simulink model "simulation_upgrade"  (R2024b)
settings: Solver=ode1be  StartTime=0.0  StopTime=10  FixedStep=0.001  RelTol=1e-3
model workspace (MAT data in the model file):
  AMP = 1
  FREQ = 1
  i_abc = 1
values from neighbouring files (symbols this model uses):
  v_WLTP = [0 0 0 0 0 0 0 0 0 0 0 0 ... (180001 elements, 1x180001)]    [v_WLTP.mat]
undefined symbols (not defined in the file or in its folder): A, a_sig, b_sig, C1, C2, C3, Cd, CG_z, downshift, Drive_wheel, Driveshaft, f_blend, f_OVD, fo, front_seat_dist, fs, g, Gearbox, i, i_sig, Inclination, Inertia, Jr2, K, m, M_curve_1, M_curve_2, m_driver, M_N_1, M_N_2, mi_c, mi_s, Mode, N_clutch, n_curve_1, n_curve_2, n_driver, n_max_1, n_max_2, n_shift, n_surfaces, Pl, Planetary, r_eq_clutch, r_geom, r_wheel, rho, Shaft, shift_time, sigma0, sigma1, sigma2, slope_angle, Stage1, Stage2, Stage3, upshift, v0, vel_wind, vs ... (+5)
libraries: simulink x29, slpidlib x3
(part 8 of 9)

== system simulation_upgrade/DRIVETRAIN/Transmission/Gearbox/DCT/Clutch1 ==
  M_in : Inport
  clutch1 : Inport  Port=2
  clutch2 : Inport  Port=3
  w_out1 : Inport  Port=4
  w_out2 : Inport  Port=5
  Clutch1 : Subsystem
      settings: PortSchema="{\"entries\":[{\"content\":{\"sides\":[{\"content\":{\"connectorIds\":[\"In1\"]},\"type\":\"ConnectorPlacement.EquallySpacedRectSide\",\"uuid\":\"a26f5a32-9f9c-4306-b7a8-6355090a4a86\"},{\"content\":{\"connectorIds\":[\"Out1\"],\"side\":\"RIGHT\"},\"type\":\"ConnectorPlacement.EquallySpacedRectSide\",\"uuid\":\"4fa489e2-cd1d-4a36-b0cb-261100046200\"},{\"content\":{\"connectorIds\":[\"In2\"],\"side\":\"TOP\"},\"type\":\"ConnectorPlacement.EquallySpacedRectSide\",\"uuid\":\"0e05a540-d6e3-4351-9a32-83f6c32571ff\"}]},\"type\":\"ConnectorPlacement.EquallySpacedConnector\",\"uuid\":\"492e0439-728a-4999-b29b-e2639b0e762e\"}],\"packageUris\":[\"http://schema.mathworks.com/mf0/Connector/R2020b\"],\"version\":\"1.0\"}"
  Clutch2 : Subsystem
      settings: PortSchema="{\"entries\":[{\"content\":{\"sides\":[{\"content\":{\"connectorIds\":[\"In1\"]},\"type\":\"ConnectorPlacement.EquallySpacedRectSide\",\"uuid\":\"a26f5a32-9f9c-4306-b7a8-6355090a4a86\"},{\"content\":{\"connectorIds\":[\"Out1\"],\"side\":\"RIGHT\"},\"type\":\"ConnectorPlacement.EquallySpacedRectSide\",\"uuid\":\"4fa489e2-cd1d-4a36-b0cb-261100046200\"},{\"content\":{\"connectorIds\":[\"In2\"],\"side\":\"TOP\"},\"type\":\"ConnectorPlacement.EquallySpacedRectSide\",\"uuid\":\"0e05a540-d6e3-4351-9a32-83f6c32571ff\"}]},\"type\":\"ConnectorPlacement.EquallySpacedConnector\",\"uuid\":\"492e0439-728a-4999-b29b-e2639b0e762e\"}],\"packageUris\":[\"http://schema.mathworks.com/mf0/Connector/R2020b\"],\"version\":\"1.0\"}"
  Constant1 : Constant  Value=2*Shaft.J+Stage2.Spur11.J+Stage2.Spur21.J
  Constant2 : Constant  Value=N_clutch*mi_s*r_eq_clutch*n_surfaces
  Divide : Product  Inputs=*/
  Integrator : Integrator
  Scope : Scope  NumInputPorts=3
  Scope1 : Scope  NumInputPorts=4
  Scope2 : Scope  NumInputPorts=3
  Scope4 : Scope  NumInputPorts=2
  Sum1 : Sum  Inputs=-+-
  Sum2 : Sum  Inputs=|+-
  Sum3 : Sum  Inputs=-+|
  M_clutch1 : Outport
  M_clutch2 : Outport  Port=2
  w_in : Outport  Port=3
  wires:
  Constant2/1 -> Scope1/4
  Sum3/1 -> Clutch1/1(delta_w), Scope2/1  "delta_w1"
  M_in/1 -> Sum1/2, Scope1/3
  w_out1/1 -> Scope2/3, Sum3/1
  Clutch1/1(M_clutch) -> M_clutch1/1, Scope1/1, Sum1/1
  Sum1/1 -> Scope4/1, Divide/1
  clutch1/1 -> Clutch1/2(" ")
  Integrator/1 -> w_in/1, Scope/2, Sum2/1, Scope2/2, Sum3/2
  Clutch2/1(M_clutch) -> Scope1/2, Sum1/3, M_clutch2/1
  clutch2/1 -> Clutch2/2(" ")
  w_out2/1 -> Scope/1, Sum2/2
  Sum2/1 -> Clutch2/1(delta_w), Scope/3  "delta_w2"
  Divide/1 -> Scope4/2, Integrator/1
  Constant1/1 -> Divide/2

== system simulation_upgrade/DRIVETRAIN/Transmission/Gearbox/DCT/Stage_2.1 ==
  note: 1) Add Subsystem or Model blocks as valid variant choices.
      | 2) You cannot connect blocks at this level. At simulation, connectivity is automatically
      | determined, based on the active variant and port name matching.
  Torque_in : Inport
  Speed_fdbk : Inport  Port=2
  Nothing : Subsystem  VariantControl=Stage2.Type == 0
  Spur : Subsystem  VariantControl=Stage2.Type == 1
  Torque_out : Outport
  Speed_out : Outport  Port=2

== system simulation_upgrade/DRIVETRAIN/Transmission/Gearbox/DCT/Stage_2.2 ==
  note: 1) Add Subsystem or Model blocks as valid variant choices.
      | 2) You cannot connect blocks at this level. At simulation, connectivity is automatically
      | determined, based on the active variant and port name matching.
  Torque_in : Inport
  Speed_fdbk : Inport  Port=2
  Nothing : Subsystem  VariantControl=Stage2.Type == 0
  Spur : Subsystem  VariantControl=Stage2.Type == 1
  Torque_out : Outport
  Speed_out : Outport  Port=2

== system simulation_upgrade/DRIVETRAIN/Transmission/Gearbox/DCT/Stage_3 ==
  note: 1) Add Subsystem or Model blocks as valid variant choices.
      | 2) You cannot connect blocks at this level. At simulation, connectivity is automatically
      | determined, based on the active variant and port name matching.
  Torque_in : Inport
  Speed_fdbk : Inport  Port=2
  Nothing : Subsystem  VariantControl=Stage3.Type == 0
  Spur : Subsystem  VariantControl=Stage3.Type == 1
  Torque_out : Outport
  Speed_out : Outport  Port=2

== system simulation_upgrade/DRIVETRAIN/Transmission/Gearbox/DCT/Triggered Subsystem ==
  In1 : Inport
  Trigger : TriggerPort  TriggerType=either  VariantControl=(inherit)  InitialTriggerSignalState=zero
  Out1 : Outport
  wires:
  In1/1 -> Out1/1

== system simulation_upgrade/DRIVETRAIN/Transmission/Gearbox/TDT/Shaft ==
  Torque_in : Inport
  Speed_fdbk : Inport  Port=2
  Derivative : Derivative
  Gain3 : Gain  Gain=J
  Sum1 : Sum  Inputs=|+-
  Torque_out : Outport
  phi_dot : Outport  Port=2
  wires:
  Speed_fdbk/1 -> phi_dot/1, Derivative/1
  Sum1/1 -> Torque_out/1
  Derivative/1 -> Gain3/1
  Gain3/1 -> Sum1/2
  Torque_in/1 -> Sum1/1

== system simulation_upgrade/DRIVETRAIN/Transmission/Gearbox/TDT/Spur ==
  Torque_in : Inport
  Speed_fdbk : Inport  Port=2
  Derivative : Derivative
  Derivative1 : Derivative
  Gain : Gain  Gain=i
  Gain2 : Gain  Gain=J2
  Gain3 : Gain  Gain=J1
  Gain4 : Gain  Gain=i
  Sum1 : Sum  Inputs=|+-
  Sum2 : Sum  Inputs=|+-
  Torque_out : Outport
  phi_dot : Outport  Port=2
  wires:
  Gain/1 -> Sum2/1
  Sum2/1 -> Torque_out/1
  Gain3/1 -> Sum1/2
  Torque_in/1 -> Sum1/1
  Gain4/1 -> Derivative1/1, phi_dot/1
  Speed_fdbk/1 -> Gain4/1, Derivative/1
  Gain2/1 -> Sum2/2
  Sum1/1 -> Gain/1
  Derivative1/1 -> Gain3/1
  Derivative/1 -> Gain2/1

== system simulation_upgrade/DRIVETRAIN/Transmission/Gearbox/TDT/Spur2 ==
  Torque_in : Inport
  Speed_fdbk : Inport  Port=2
  Derivative : Derivative
  Derivative1 : Derivative
  Gain : Gain  Gain=i
  Gain2 : Gain  Gain=J2
  Gain3 : Gain  Gain=J1
  Gain4 : Gain  Gain=i
  Sum1 : Sum  Inputs=|+-
  Sum2 : Sum  Inputs=|+-
  Torque_out : Outport
  phi_dot : Outport  Port=2
  wires:
  Derivative/1 -> Gain2/1
  Derivative1/1 -> Gain3/1
  Sum1/1 -> Gain/1
  Gain2/1 -> Sum2/2
  Speed_fdbk/1 -> Derivative/1, Gain4/1
  Gain4/1 -> phi_dot/1, Derivative1/1
  Torque_in/1 -> Sum1/1
  Gain3/1 -> Sum1/2
  Sum2/1 -> Torque_out/1
  Gain/1 -> Sum2/1

== system simulation_upgrade/DRIVETRAIN/Transmission/Gearbox/TDT/Stage_1 ==
  note: 1) Add Subsystem or Model blocks as valid variant choices.
      | 2) You cannot connect blocks at this level. At simulation, connectivity is automatically
      | determined, based on the active variant and port name matching.
  Torque_in : Inport
  Speed_fdbk : Inport  Port=2
  Nothing : Subsystem  VariantControl=Stage1.Type == 0
  Spur : Subsystem  VariantControl=Stage1.Type == 1
  Torque_out : Outport
  Speed_out : Outport  Port=2

== system simulation_upgrade/DRIVETRAIN/Transmission/Gearbox/TDT/Stage_2.1 ==
  note: 1) Add Subsystem or Model blocks as valid variant choices.
      | 2) You cannot connect blocks at this level. At simulation, connectivity is automatically
      | determined, based on the active variant and port name matching.
  Torque_in : Inport
  Speed_fdbk : Inport  Port=2
  Nothing : Subsystem  VariantControl=Stage2.Type == 0
  Spur : Subsystem  VariantControl=Stage2.Type == 1
  Torque_out : Outport
  Speed_out : Outport  Port=2

== system simulation_upgrade/DRIVETRAIN/Transmission/Gearbox/TDT/Stage_2.2 ==
  note: 1) Add Subsystem or Model blocks as valid variant choices.
      | 2) You cannot connect blocks at this level. At simulation, connectivity is automatically
      | determined, based on the active variant and port name matching.
  Torque_in : Inport
  Speed_fdbk : Inport  Port=2
  Nothing : Subsystem  VariantControl=Stage2.Type == 0
  Spur : Subsystem  VariantControl=Stage2.Type == 1
  Torque_out : Outport
  Speed_out : Outport  Port=2

== system simulation_upgrade/DRIVETRAIN/Transmission/Gearbox/TDT/Stage_3 ==
  note: 1) Add Subsystem or Model blocks as valid variant choices.
      | 2) You cannot connect blocks at this level. At simulation, connectivity is automatically
      | determined, based on the active variant and port name matching.
  Torque_in : Inport
  Speed_fdbk : Inport  Port=2
  Nothing : Subsystem  VariantControl=Stage3.Type == 0
  Spur : Subsystem  VariantControl=Stage3.Type == 1
  Torque_out : Outport
  Speed_out : Outport  Port=2

== system simulation_upgrade/DRIVETRAIN/Transmission/Gearbox/TDT/Subsystem ==
  Spur 21 : Inport
  Spur22 : Inport  Port=2
  Multiport Switch : MultiPortSwitch  DataPortOrder=Zero-based contiguous  Inputs=8  zeroidx=on  SaturateOnIntegerOverflow=off  InputSameDT=off
  Multiport Switch1 : MultiPortSwitch  DataPortOrder=Zero-based contiguous  zeroidx=on  SaturateOnIntegerOverflow=off  InputSameDT=off
  Switch : Switch  Criteria=u2 > Threshold  Threshold=1  SaturateOnIntegerOverflow=off  InputSameDT=off
  Switch1 : Switch  Criteria=u2 > Threshold  Threshold=1  SaturateOnIntegerOverflow=off  InputSameDT=off
  Out : Outport
  wires:
  Multiport Switch/1 -> Out/1
  [Gear] -> Multiport Switch1/1
  Spur 21/1 -> Multiport Switch1/3, Switch1/1, Switch/3
  Spur22/1 -> Switch/1, Switch1/3, Multiport Switch1/4
  Multiport Switch1/1 -> Multiport Switch/9, Multiport Switch/8, Multiport Switch/7, Multiport Switch/4, Multiport Switch/3, Multiport Switch/2
  [shifting_stage] -> Multiport Switch/1
  [GearSet] -> Switch/2, Switch1/2
  Switch/1 -> Multiport Switch1/2, Multiport Switch/6
  Switch1/1 -> Multiport Switch/5

== system simulation_upgrade/PANEL/Pretty shot/Transmission /Variant Subsystem/Automated Manual Transmission ==
  " " : Inport
  "  " : Outport

== system simulation_upgrade/PANEL/Pretty shot/Transmission /Variant Subsystem/Automatic Transmission ==
  " " : Inport
  "  " : Outport

== system simulation_upgrade/PANEL/Pretty shot/Transmission /Variant Subsystem/Twin Drive Transmission ==
  " " : Inport
  To Workspace : ToWorkspace  VariableName=v_TDT1  SaveFormat=Timeseries  SampleTime=-1
  To Workspace1 : ToWorkspace  VariableName=acc_TDT1  SaveFormat=Timeseries  SampleTime=-1
  To Workspace2 : ToWorkspace  VariableName=jerk_TDT1  SaveFormat=Timeseries  SampleTime=-1
  "  " : Outport
  wires:
  " "/1 -> "  "/1
  [Speed] -> To Workspace/1
  [acc] -> To Workspace1/1
  [jerk] -> To Workspace2/1

== system simulation_upgrade/CONTROLS/Main Control Unit/AT_MCU/Clutch_Profile/polynomial_s_response/signal_register ==
  signal : Inport
  Trigger : TriggerPort  TriggerType=either  VariantControl=(inherit)  PortDimensions=1
  Memory : Memory  InheritSampleTime=on
  Subtract : Sum  Inputs=+-
  previous_value : Outport
  difference : Outport  Port=2
  wires:
  signal/1 -> Memory/1, Subtract/1
  Memory/1 -> previous_value/1, Subtract/2
  Subtract/1 -> difference/1

== system simulation_upgrade/CONTROLS/Main Control Unit/AT_MCU/Clutch_Profile/polynomial_s_response/time_register ==
  t : Inport
  Trigger : TriggerPort  TriggerType=either  VariantControl=(inherit)  PortDimensions=1
  t0 : Outport
  wires:
  t/1 -> t0/1

== system simulation_upgrade/CONTROLS/Main Control Unit/AT_MCU/Clutch_Profile/polynomial_s_response1/signal_register ==
  signal : Inport
  Trigger : TriggerPort  TriggerType=either  VariantControl=(inherit)  PortDimensions=1
  Memory : Memory  InheritSampleTime=on
  Subtract : Sum  Inputs=+-
  previous_value : Outport
  difference : Outport  Port=2
  wires:
  Subtract/1 -> difference/1
  Memory/1 -> Subtract/2, previous_value/1
  signal/1 -> Subtract/1, Memory/1

== system simulation_upgrade/CONTROLS/Main Control Unit/AT_MCU/Clutch_Profile/polynomial_s_response1/time_register ==
  t : Inport
  Trigger : TriggerPort  TriggerType=either  VariantControl=(inherit)  PortDimensions=1
  t0 : Outport
  wires:
  t/1 -> t0/1

== system simulation_upgrade/CONTROLS/Main Control Unit/AT_MCU/Clutch_Profile/sigmoid_response/signal_register ==
  signal : Inport
  Trigger : TriggerPort  TriggerType=either  VariantControl=(inherit)  PortDimensions=1
  Delay : Delay  DelayLength=1  InputProcessing=Columns as channels (frame based)
  Subtract : Sum  Inputs=+-
  previous_value : Outport
  difference : Outport  Port=2
  wires:
  signal/1 -> Delay/1, Subtract/1
  Delay/1 -> previous_value/1, Subtract/2
  Subtract/1 -> difference/1

== system simulation_upgrade/CONTROLS/Main Control Unit/AT_MCU/Clutch_Profile/sigmoid_response/time_register ==
  t : Inport
  Trigger : TriggerPort  TriggerType=either  VariantControl=(inherit)  PortDimensions=1
  t0 : Outport
  wires:
  t/1 -> t0/1

== system simulation_upgrade/CONTROLS/Main Control Unit/AT_MCU/Clutch_Profile/sigmoid_response1/signal_register ==
  signal : Inport
  Trigger : TriggerPort  TriggerType=either  VariantControl=(inherit)  PortDimensions=1
  Delay : Delay  DelayLength=1  InputProcessing=Columns as channels (frame based)
  Subtract : Sum  Inputs=+-
  previous_value : Outport
  difference : Outport  Port=2
  wires:
  Subtract/1 -> difference/1
  Delay/1 -> Subtract/2, previous_value/1
  signal/1 -> Subtract/1, Delay/1

== system simulation_upgrade/CONTROLS/Main Control Unit/AT_MCU/Clutch_Profile/sigmoid_response1/time_register ==
  t : Inport
  Trigger : TriggerPort  TriggerType=either  VariantControl=(inherit)  PortDimensions=1
  t0 : Outport
  wires:
  t/1 -> t0/1

== system simulation_upgrade/DRIVETRAIN/Transmission/Gearbox/AMT/Clutch/Clutch1 ==
  delta_w : Inport
  " " : Inport  Port=2
  Gain10 : Gain  Gain=r_eq_clutch
  Gain3 : Gain  Gain=r_eq_clutch
  Scope2 : Scope  NumInputPorts=2
  Scope3 : Scope
  Subsystem : Subsystem
      settings: PortSchema="{\"entries\":[{\"content\":{\"sides\":[{\"content\":{\"connectorIds\":[\"In1\"]},\"type\":\"ConnectorPlacement.EquallySpacedRectSide\",\"uuid\":\"0ae2ed28-5be6-4ce0-b87c-2c13a72d1ad0\"},{\"content\":{\"connectorIds\":[\"In2\",\"Out1\"],\"side\":\"RIGHT\"},\"type\":\"ConnectorPlacement.EquallySpacedRectSide\",\"uuid\":\"8d48d664-ebaf-4c3e-be9e-f793543e8061\"},{\"content\":{\"side\":\"TOP\"},\"type\":\"ConnectorPlacement.EquallySpacedRectSide\",\"uuid\":\"2d66836a-de46-4974-a48b-ee2778be1c08\"},{\"content\":{\"side\":\"BOTTOM\"},\"type\":\"ConnectorPlacement.EquallySpacedRectSide\",\"uuid\":\"e232d9f4-6257-4976-8384-26c462ae0041\"}]},\"type\":\"ConnectorPlacement.EquallySpacedConnector\",\"uuid\":\"ae24f926-3a59-4a74-9cf0-af55dcfbad19\"}],\"packageUris\":[\"http://schema.mathworks.com/mf0/Connector/R2020b\"],\"version\":\"1.0\"}"
      mask Display: image('images/Stribeck.png');
  Subsystem1 : Subsystem
      settings: PortSchema="{\"entries\":[{\"content\":{\"sides\":[{\"content\":{\"connectorIds\":[\"In1\",\"In2\"]},\"type\":\"ConnectorPlacement.EquallySpacedRectSide\",\"uuid\":\"9e2cbd08-5b8a-4c75-ae53-c0d295cfe494\"},{\"content\":{\"connectorIds\":[\"Out1\",\"Out2\"],\"side\":\"RIGHT\"},\"type\":\"ConnectorPlacement.EquallySpacedRectSide\",\"uuid\":\"77a3a6f0-22a7-43a6-8d61-33ee07a6a335\"},{\"content\":{\"side\":\"TOP\"},\"type\":\"ConnectorPlacement.EquallySpacedRectSide\",\"uuid\":\"42262743-4dc6-4297-a012-95f629a18d23\"},{\"content\":{\"connectorIds\":[\"In3\"],\"side\":\"BOTTOM\"},\"type\":\"ConnectorPlacement.EquallySpacedRectSide\",\"uuid\":\"a89123f6-acee-411d-93c1-3b5d847486f5\"}]},\"type\":\"ConnectorPlacement.EquallySpacedConnector\",\"uuid\":\"ae5ede95-cba8-4d2e-b0da-ab555bd567a9\"}],\"packageUris\":[\"http://schema.mathworks.com/mf0/Connector/R2020b\"],\"version\":\"1.0\"}"
      mask Display: image('images/z_state.png');
  Subsystem2 : Subsystem
      settings: PortSchema="{\"entries\":[{\"content\":{\"sides\":[{\"content\":{\"connectorIds\":[\"In1\",\"In2\",\"In3\"]},\"type\":\"ConnectorPlacement.EquallySpacedRectSide\",\"uuid\":\"1b79fb4b-1921-4665-8eba-b393f9ea98d6\"},{\"content\":{\"connectorIds\":[\"Out1\"],\"side\":\"RIGHT\"},\"type\":\"ConnectorPlacement.EquallySpacedRectSide\",\"uuid\":\"084d95ac-1716-4b0b-a696-3271535a91cf\"},{\"content\":{\"side\":\"TOP\"},\"type\":\"ConnectorPlacement.EquallySpacedRectSide\",\"uuid\":\"ec91298b-c3b0-4df1-a0b8-53c7de39a879\"},{\"content\":{\"connectorIds\":[\"In4\"],\"side\":\"BOTTOM\"},\"type\":\"ConnectorPlacement.EquallySpacedRectSide\",\"uuid\":\"de14d308-9d82-4371-86bd-ca5ab581d7ed\"}]},\"type\":\"ConnectorPlacement.EquallySpacedConnector\",\"uuid\":\"ce361a1b-48ea-4ff5-b8e2-9f4b10df6d4d\"}],\"packageUris\":[\"http://schema.mathworks.com/mf0/Connector/R2020b\"],\"version\":\"1.0\"}"
      mask Display: image('images/fric_force.png');
  M_clutch : Outport
  wires:
  delta_w/1 -> Gain3/1
  Subsystem1/2(z) -> Scope2/1, Subsystem2/3(z)
  Subsystem1/1(z_dot) -> Scope2/2, Subsystem2/2(z_dot)
  Subsystem2/1(F) -> Gain10/1
  Gain10/1 -> M_clutch/1  "M_clutch"
  Gain3/1 -> Scope3/1, Subsystem2/1(v), Subsystem/2(v), Subsystem1/1(v)  "v"
  " "/1 -> Subsystem2/4(" "), Subsystem1/3(In1), Subsystem/1(N)
  Subsystem/1(g(v)) -> Subsystem1/2(g(v))

== system simulation_upgrade/DRIVETRAIN/Transmission/Gearbox/AMT/Stage_1/Nothing ==
  Torque_in : Inport
  Speed_fdbk : Inport  Port=2
  Torque_out : Outport
  Speed_out : Outport  Port=2
  wires:
  Torque_in/1 -> Torque_out/1
  Speed_fdbk/1 -> Speed_out/1

== system simulation_upgrade/DRIVETRAIN/Transmission/Gearbox/AMT/Stage_1/Spur ==
  Torque_in : Inport
  Speed_fdbk : Inport  Port=2
  Shaft1 : Subsystem  mask{J=Shaft.J}
      mask prompts: J "Inertia_kgm^2"
      settings: PortSchema="{\"entries\":[{\"content\":{\"sides\":[{\"content\":{\"connectorIds\":[\"In1\",\"Out2\"]},\"type\":\"ConnectorPlacement.EquallySpacedRectSide\",\"uuid\":\"898fedf9-82f7-4bc2-bf05-880de36b191d\"},{\"content\":{\"connectorIds\":[\"Out1\",\"In2\"],\"side\":\"RIGHT\"},\"type\":\"ConnectorPlacement.EquallySpacedRectSide\",\"uuid\":\"50317b6c-245f-4bd1-a8cd-7a774957ae86\"},{\"content\":{\"side\":\"TOP\"},\"type\":\"ConnectorPlacement.EquallySpacedRectSide\",\"uuid\":\"ff1de2a1-7305-40d8-9e1f-fd0fa1e7d830\"}]},\"type\":\"ConnectorPlacement.EquallySpacedConnector\",\"uuid\":\"6ce82d73-f3da-4f59-9039-464a6ef3e9c5\"}],\"packageUris\":[\"http://schema.mathworks.com/mf0/Connector/R2020b\"],\"version\":\"1.0\"}"
  Spur1 : Subsystem  mask{i=Stage1.i, J1=Stage1.Spur1.J, J2=Stage1.Spur2.J}
      mask prompts: i "Ratio"; J1 "Input_Gear_Inertia"; J2 "Output_Gear_Inertia"
      settings: PortSchema="{\"entries\":[{\"content\":{\"sides\":[{\"content\":{\"connectorIds\":[\"In1\",\"Out2\"]},\"type\":\"ConnectorPlacement.EquallySpacedRectSide\",\"uuid\":\"898fedf9-82f7-4bc2-bf05-880de36b191d\"},{\"content\":{\"connectorIds\":[\"Out1\",\"In2\"],\"side\":\"RIGHT\"},\"type\":\"ConnectorPlacement.EquallySpacedRectSide\",\"uuid\":\"50317b6c-245f-4bd1-a8cd-7a774957ae86\"},{\"content\":{\"side\":\"TOP\"},\"type\":\"ConnectorPlacement.EquallySpacedRectSide\",\"uuid\":\"ff1de2a1-7305-40d8-9e1f-fd0fa1e7d830\"}]},\"type\":\"ConnectorPlacement.EquallySpacedConnector\",\"uuid\":\"6ce82d73-f3da-4f59-9039-464a6ef3e9c5\"}],\"packageUris\":[\"http://schema.mathworks.com/mf0/Connector/R2020b\"],\"version\":\"1.0\"}"
  Torque_out : Outport
  Speed_out : Outport  Port=2
  wires:
  Speed_fdbk/1 -> Shaft1/2(Speed_fdbk)
  Torque_in/1 -> Spur1/1(Torque_in)  "T_Rotor"
  Shaft1/1(Torque_out) -> Torque_out/1  "T_Gear_2"
  Spur1/2(phi_dot) -> Speed_out/1
  Shaft1/2(phi_dot) -> Spur1/2(Speed_fdbk)
  Spur1/1(Torque_out) -> Shaft1/1(Torque_in)

== system simulation_upgrade/DRIVETRAIN/Transmission/Gearbox/AMT/Stage_2.1/Nothing ==
  Torque_in : Inport
  Speed_fdbk : Inport  Port=2
  Torque_out : Outport
  Speed_out : Outport  Port=2
  wires:
  Torque_in/1 -> Torque_out/1  "T_Rotor"
  Speed_fdbk/1 -> Speed_out/1

== system simulation_upgrade/DRIVETRAIN/Transmission/Gearbox/AMT/Stage_2.1/Spur ==
  Torque_in : Inport
  Speed_fdbk : Inport  Port=2
  Spur2 : Subsystem  mask{i=Stage2.i1, J1=Stage2.Spur11.J, J2=Stage2.Spur12.J}
      mask prompts: i "Ratio"; J1 "Input_Gear_Inertia"; J2 "Output_Gear_Inertia"
      settings: PortSchema="{\"entries\":[{\"content\":{\"sides\":[{\"content\":{\"connectorIds\":[\"In1\",\"Out2\"]},\"type\":\"ConnectorPlacement.EquallySpacedRectSide\",\"uuid\":\"898fedf9-82f7-4bc2-bf05-880de36b191d\"},{\"content\":{\"connectorIds\":[\"Out1\",\"In2\"],\"side\":\"RIGHT\"},\"type\":\"ConnectorPlacement.EquallySpacedRectSide\",\"uuid\":\"50317b6c-245f-4bd1-a8cd-7a774957ae86\"},{\"content\":{\"side\":\"TOP\"},\"type\":\"ConnectorPlacement.EquallySpacedRectSide\",\"uuid\":\"ff1de2a1-7305-40d8-9e1f-fd0fa1e7d830\"}]},\"type\":\"ConnectorPlacement.EquallySpacedConnector\",\"uuid\":\"6ce82d73-f3da-4f59-9039-464a6ef3e9c5\"}],\"packageUris\":[\"http://schema.mathworks.com/mf0/Connector/R2020b\"],\"version\":\"1.0\"}"
  Torque_out : Outport
  Speed_out : Outport  Port=2
  wires:
  Speed_fdbk/1 -> Spur2/2(Speed_fdbk)
  Torque_in/1 -> Spur2/1(Torque_in)
  Spur2/2(phi_dot) -> Speed_out/1
  Spur2/1(Torque_out) -> Torque_out/1

== system simulation_upgrade/DRIVETRAIN/Transmission/Gearbox/AMT/Stage_2.2/Nothing ==
  Torque_in : Inport
  Speed_fdbk : Inport  Port=2
  Torque_out : Outport
  Speed_out : Outport  Port=2
  wires:
  Torque_in/1 -> Torque_out/1  "T_Rotor"
  Speed_fdbk/1 -> Speed_out/1

== system simulation_upgrade/DRIVETRAIN/Transmission/Gearbox/AMT/Stage_2.2/Spur ==
  Torque_in : Inport
  Speed_fdbk : Inport  Port=2
  Spur2 : Subsystem  mask{i=Stage2.i2, J1=Stage2.Spur21.J, J2=Stage2.Spur22.J}
      mask prompts: i "Ratio"; J1 "Input_Gear_Inertia"; J2 "Output_Gear_Inertia"
      settings: PortSchema="{\"entries\":[{\"content\":{\"sides\":[{\"content\":{\"connectorIds\":[\"In1\",\"Out2\"]},\"type\":\"ConnectorPlacement.EquallySpacedRectSide\",\"uuid\":\"898fedf9-82f7-4bc2-bf05-880de36b191d\"},{\"content\":{\"connectorIds\":[\"Out1\",\"In2\"],\"side\":\"RIGHT\"},\"type\":\"ConnectorPlacement.EquallySpacedRectSide\",\"uuid\":\"50317b6c-245f-4bd1-a8cd-7a774957ae86\"},{\"content\":{\"side\":\"TOP\"},\"type\":\"ConnectorPlacement.EquallySpacedRectSide\",\"uuid\":\"ff1de2a1-7305-40d8-9e1f-fd0fa1e7d830\"}]},\"type\":\"ConnectorPlacement.EquallySpacedConnector\",\"uuid\":\"6ce82d73-f3da-4f59-9039-464a6ef3e9c5\"}],\"packageUris\":[\"http://schema.mathworks.com/mf0/Connector/R2020b\"],\"version\":\"1.0\"}"
  Torque_out : Outport
  Speed_out : Outport  Port=2
  wires:
  Torque_in/1 -> Spur2/1(Torque_in)
  Spur2/2(phi_dot) -> Speed_out/1
  Spur2/1(Torque_out) -> Torque_out/1
  Speed_fdbk/1 -> Spur2/2(Speed_fdbk)

== system simulation_upgrade/DRIVETRAIN/Transmission/Gearbox/AMT/Stage_3/Nothing ==
  Torque_in : Inport
  Speed_fdbk : Inport  Port=2
  Torque_out : Outport
  Speed_out : Outport  Port=2
  wires:
  Speed_fdbk/1 -> Speed_out/1
  Torque_in/1 -> Torque_out/1

== system simulation_upgrade/DRIVETRAIN/Transmission/Gearbox/AMT/Stage_3/Spur ==
  Torque_in : Inport
  Speed_fdbk : Inport  Port=2
  Shaft : Subsystem  mask{J=Shaft.J}
      mask prompts: J "Inertia_kgm^2"
      settings: PortSchema="{\"entries\":[{\"content\":{\"sides\":[{\"content\":{\"connectorIds\":[\"In1\",\"Out2\"]},\"type\":\"ConnectorPlacement.EquallySpacedRectSide\",\"uuid\":\"898fedf9-82f7-4bc2-bf05-880de36b191d\"},{\"content\":{\"connectorIds\":[\"Out1\",\"In2\"],\"side\":\"RIGHT\"},\"type\":\"ConnectorPlacement.EquallySpacedRectSide\",\"uuid\":\"50317b6c-245f-4bd1-a8cd-7a774957ae86\"},{\"content\":{\"side\":\"TOP\"},\"type\":\"ConnectorPlacement.EquallySpacedRectSide\",\"uuid\":\"ff1de2a1-7305-40d8-9e1f-fd0fa1e7d830\"}]},\"type\":\"ConnectorPlacement.EquallySpacedConnector\",\"uuid\":\"6ce82d73-f3da-4f59-9039-464a6ef3e9c5\"}],\"packageUris\":[\"http://schema.mathworks.com/mf0/Connector/R2020b\"],\"version\":\"1.0\"}"
  Spur3 : Subsystem  mask{i=Stage3.i, J1=Stage3.Spur1.J, J2=Stage3.Spur2.J}
      mask prompts: i "Ratio"; J1 "Input_Gear_Inertia"; J2 "Output_Gear_Inertia"
      settings: PortSchema="{\"entries\":[{\"content\":{\"sides\":[{\"content\":{\"connectorIds\":[\"In1\",\"Out2\"]},\"type\":\"ConnectorPlacement.EquallySpacedRectSide\",\"uuid\":\"898fedf9-82f7-4bc2-bf05-880de36b191d\"},{\"content\":{\"connectorIds\":[\"Out1\",\"In2\"],\"side\":\"RIGHT\"},\"type\":\"ConnectorPlacement.EquallySpacedRectSide\",\"uuid\":\"50317b6c-245f-4bd1-a8cd-7a774957ae86\"},{\"content\":{\"side\":\"TOP\"},\"type\":\"ConnectorPlacement.EquallySpacedRectSide\",\"uuid\":\"ff1de2a1-7305-40d8-9e1f-fd0fa1e7d830\"}]},\"type\":\"ConnectorPlacement.EquallySpacedConnector\",\"uuid\":\"6ce82d73-f3da-4f59-9039-464a6ef3e9c5\"}],\"packageUris\":[\"http://schema.mathworks.com/mf0/Connector/R2020b\"],\"version\":\"1.0\"}"
  Torque_out : Outport
  Speed_out : Outport  Port=2
  wires:
  Speed_fdbk/1 -> Spur3/2(Speed_fdbk)
  Spur3/2(phi_dot) -> Shaft/2(Speed_fdbk)
  Spur3/1(Torque_out) -> Torque_out/1
  Torque_in/1 -> Shaft/1(Torque_in)
  Shaft/2(phi_dot) -> Speed_out/1
  Shaft/1(Torque_out) -> Spur3/1(Torque_in)

== system simulation_upgrade/DRIVETRAIN/Transmission/Gearbox/AT/Stage_3/Nothing ==
  Torque_in : Inport
  Speed_fdbk : Inport  Port=2
  Torque_out : Outport
  Speed_out : Outport  Port=2
  wires:
  Speed_fdbk/1 -> Speed_out/1
  Torque_in/1 -> Torque_out/1

== system simulation_upgrade/DRIVETRAIN/Transmission/Gearbox/AT/Stage_3/Spur ==
  Torque_in : Inport
  Speed_fdbk : Inport  Port=2
  Spur3 : Subsystem  mask{i=Stage3.i, J1=Stage3.Spur1.J, J2=Stage3.Spur2.J}
      mask prompts: i "Ratio"; J1 "Input_Gear_Inertia"; J2 "Output_Gear_Inertia"
      settings: PortSchema="{\"entries\":[{\"content\":{\"sides\":[{\"content\":{\"connectorIds\":[\"In1\",\"Out2\"]},\"type\":\"ConnectorPlacement.EquallySpacedRectSide\",\"uuid\":\"898fedf9-82f7-4bc2-bf05-880de36b191d\"},{\"content\":{\"connectorIds\":[\"Out1\",\"In2\"],\"side\":\"RIGHT\"},\"type\":\"ConnectorPlacement.EquallySpacedRectSide\",\"uuid\":\"50317b6c-245f-4bd1-a8cd-7a774957ae86\"},{\"content\":{\"side\":\"TOP\"},\"type\":\"ConnectorPlacement.EquallySpacedRectSide\",\"uuid\":\"ff1de2a1-7305-40d8-9e1f-fd0fa1e7d830\"}]},\"type\":\"ConnectorPlacement.EquallySpacedConnector\",\"uuid\":\"6ce82d73-f3da-4f59-9039-464a6ef3e9c5\"}],\"packageUris\":[\"http://schema.mathworks.com/mf0/Connector/R2020b\"],\"version\":\"1.0\"}"
  Torque_out : Outport
  Speed_out : Outport  Port=2
  wires:
  Speed_fdbk/1 -> Spur3/2(Speed_fdbk)
  Spur3/2(phi_dot) -> Speed_out/1
  Spur3/1(Torque_out) -> Torque_out/1
  Torque_in/1 -> Spur3/1(Torque_in)

== system simulation_upgrade/DRIVETRAIN/Transmission/Gearbox/DCT/Clutch1/Clutch1 ==
  delta_w : Inport
  " " : Inport  Port=2
  Gain10 : Gain  Gain=r_eq_clutch
  Gain3 : Gain  Gain=r_eq_clutch
  Scope2 : Scope  NumInputPorts=2
  Scope3 : Scope
  Subsystem : Subsystem
      settings: PortSchema="{\"entries\":[{\"content\":{\"sides\":[{\"content\":{\"connectorIds\":[\"In1\"]},\"type\":\"ConnectorPlacement.EquallySpacedRectSide\",\"uuid\":\"0ae2ed28-5be6-4ce0-b87c-2c13a72d1ad0\"},{\"content\":{\"connectorIds\":[\"In2\",\"Out1\"],\"side\":\"RIGHT\"},\"type\":\"ConnectorPlacement.EquallySpacedRectSide\",\"uuid\":\"8d48d664-ebaf-4c3e-be9e-f793543e8061\"},{\"content\":{\"side\":\"TOP\"},\"type\":\"ConnectorPlacement.EquallySpacedRectSide\",\"uuid\":\"2d66836a-de46-4974-a48b-ee2778be1c08\"},{\"content\":{\"side\":\"BOTTOM\"},\"type\":\"ConnectorPlacement.EquallySpacedRectSide\",\"uuid\":\"e232d9f4-6257-4976-8384-26c462ae0041\"}]},\"type\":\"ConnectorPlacement.EquallySpacedConnector\",\"uuid\":\"ae24f926-3a59-4a74-9cf0-af55dcfbad19\"}],\"packageUris\":[\"http://schema.mathworks.com/mf0/Connector/R2020b\"],\"version\":\"1.0\"}"
      mask Display: image('images/Stribeck.png');
  Subsystem1 : Subsystem
      settings: PortSchema="{\"entries\":[{\"content\":{\"sides\":[{\"content\":{\"connectorIds\":[\"In1\",\"In2\"]},\"type\":\"ConnectorPlacement.EquallySpacedRectSide\",\"uuid\":\"fba00446-fe01-4fd0-a740-7d5efbf0abc7\"},{\"content\":{\"connectorIds\":[\"Out1\",\"Out2\"],\"side\":\"RIGHT\"},\"type\":\"ConnectorPlacement.EquallySpacedRectSide\",\"uuid\":\"28d31996-59d3-4656-988b-c785e0d07c46\"},{\"content\":{\"side\":\"TOP\"},\"type\":\"ConnectorPlacement.EquallySpacedRectSide\",\"uuid\":\"07dfb693-bdac-419f-bf8c-22f11bb5a1ff\"},{\"content\":{\"connectorIds\":[\"In3\"],\"side\":\"BOTTOM\"},\"type\":\"ConnectorPlacement.EquallySpacedRectSide\",\"uuid\":\"e46b7f0d-22dc-4b01-9fc3-2183fe5bd14e\"}]},\"type\":\"ConnectorPlacement.EquallySpacedConnector\",\"uuid\":\"53afe5e8-6f41-4676-b5a4-a094561728b0\"}],\"packageUris\":[\"http://schema.mathworks.com/mf0/Connector/R2020b\"],\"version\":\"1.0\"}"
      mask Display: image('images/z_state.png');
  Subsystem2 : Subsystem
      settings: PortSchema="{\"entries\":[{\"content\":{\"sides\":[{\"content\":{\"connectorIds\":[\"In1\",\"In2\",\"In3\"]},\"type\":\"ConnectorPlacement.EquallySpacedRectSide\",\"uuid\":\"718e9a4c-012a-432e-af1d-56a8c510a1ff\"},{\"content\":{\"connectorIds\":[\"Out1\"],\"side\":\"RIGHT\"},\"type\":\"ConnectorPlacement.EquallySpacedRectSide\",\"uuid\":\"b8acef94-ef29-40e0-b6df-913e21cb4db2\"},{\"content\":{\"side\":\"TOP\"},\"type\":\"ConnectorPlacement.EquallySpacedRectSide\",\"uuid\":\"42ba6916-bf07-457b-89e7-b10a87e70d96\"},{\"content\":{\"connectorIds\":[\"In4\"],\"side\":\"BOTTOM\"},\"type\":\"ConnectorPlacement.EquallySpacedRectSide\",\"uuid\":\"25c3a005-357f-4967-9fb3-686ba180841f\"}]},\"type\":\"ConnectorPlacement.EquallySpacedConnector\",\"uuid\":\"db3b50fc-f4cd-400b-b8f7-b0301a8ba65b\"}],\"packageUris\":[\"http://schema.mathworks.com/mf0/Connector/R2020b\"],\"version\":\"1.0\"}"
      mask Display: image('images/fric_force.png');
  M_clutch : Outport
  wires:
  delta_w/1 -> Gain3/1
  Subsystem1/2(z) -> Scope2/1, Subsystem2/3(z)
  Subsystem1/1(z_dot) -> Scope2/2, Subsystem2/2(z_dot)
  Subsystem2/1(F) -> Gain10/1
  Gain10/1 -> M_clutch/1  "M_clutch"
  Gain3/1 -> Scope3/1, Subsystem2/1(v), Subsystem1/1(v), Subsystem/2(v)  "v"
  Subsystem/1(g(v)) -> Subsystem1/2(g(v))
  " "/1 -> Subsystem2/4(" "), Subsystem1/3(" "), Subsystem/1(N)

== system simulation_upgrade/DRIVETRAIN/Transmission/Gearbox/DCT/Clutch1/Clutch2 ==
  delta_w : Inport
  " " : Inport  Port=2
  Gain10 : Gain  Gain=r_eq_clutch
  Gain3 : Gain  Gain=r_eq_clutch
  Scope2 : Scope  NumInputPorts=2
  Scope3 : Scope
  Subsystem : Subsystem
      settings: PortSchema="{\"entries\":[{\"content\":{\"sides\":[{\"content\":{\"connectorIds\":[\"In1\"]},\"type\":\"ConnectorPlacement.EquallySpacedRectSide\",\"uuid\":\"0ae2ed28-5be6-4ce0-b87c-2c13a72d1ad0\"},{\"content\":{\"connectorIds\":[\"In2\",\"Out1\"],\"side\":\"RIGHT\"},\"type\":\"ConnectorPlacement.EquallySpacedRectSide\",\"uuid\":\"8d48d664-ebaf-4c3e-be9e-f793543e8061\"},{\"content\":{\"side\":\"TOP\"},\"type\":\"ConnectorPlacement.EquallySpacedRectSide\",\"uuid\":\"2d66836a-de46-4974-a48b-ee2778be1c08\"},{\"content\":{\"side\":\"BOTTOM\"},\"type\":\"ConnectorPlacement.EquallySpacedRectSide\",\"uuid\":\"e232d9f4-6257-4976-8384-26c462ae0041\"}]},\"type\":\"ConnectorPlacement.EquallySpacedConnector\",\"uuid\":\"ae24f926-3a59-4a74-9cf0-af55dcfbad19\"}],\"packageUris\":[\"http://schema.mathworks.com/mf0/Connector/R2020b\"],\"version\":\"1.0\"}"
      mask Display: image('images/Stribeck.png');
  Subsystem1 : Subsystem
      settings: PortSchema="{\"entries\":[{\"content\":{\"sides\":[{\"content\":{\"connectorIds\":[\"In1\",\"In2\"]},\"type\":\"ConnectorPlacement.EquallySpacedRectSide\",\"uuid\":\"fba00446-fe01-4fd0-a740-7d5efbf0abc7\"},{\"content\":{\"connectorIds\":[\"Out1\",\"Out2\"],\"side\":\"RIGHT\"},\"type\":\"ConnectorPlacement.EquallySpacedRectSide\",\"uuid\":\"28d31996-59d3-4656-988b-c785e0d07c46\"},{\"content\":{\"side\":\"TOP\"},\"type\":\"ConnectorPlacement.EquallySpacedRectSide\",\"uuid\":\"07dfb693-bdac-419f-bf8c-22f11bb5a1ff\"},{\"content\":{\"connectorIds\":[\"In3\"],\"side\":\"BOTTOM\"},\"type\":\"ConnectorPlacement.EquallySpacedRectSide\",\"uuid\":\"e46b7f0d-22dc-4b01-9fc3-2183fe5bd14e\"}]},\"type\":\"ConnectorPlacement.EquallySpacedConnector\",\"uuid\":\"53afe5e8-6f41-4676-b5a4-a094561728b0\"}],\"packageUris\":[\"http://schema.mathworks.com/mf0/Connector/R2020b\"],\"version\":\"1.0\"}"
      mask Display: image('images/z_state.png');
  Subsystem2 : Subsystem
      settings: PortSchema="{\"entries\":[{\"content\":{\"sides\":[{\"content\":{\"connectorIds\":[\"In1\",\"In2\",\"In3\"]},\"type\":\"ConnectorPlacement.EquallySpacedRectSide\",\"uuid\":\"718e9a4c-012a-432e-af1d-56a8c510a1ff\"},{\"content\":{\"connectorIds\":[\"Out1\"],\"side\":\"RIGHT\"},\"type\":\"ConnectorPlacement.EquallySpacedRectSide\",\"uuid\":\"b8acef94-ef29-40e0-b6df-913e21cb4db2\"},{\"content\":{\"side\":\"TOP\"},\"type\":\"ConnectorPlacement.EquallySpacedRectSide\",\"uuid\":\"42ba6916-bf07-457b-89e7-b10a87e70d96\"},{\"content\":{\"connectorIds\":[\"In4\"],\"side\":\"BOTTOM\"},\"type\":\"ConnectorPlacement.EquallySpacedRectSide\",\"uuid\":\"25c3a005-357f-4967-9fb3-686ba180841f\"}]},\"type\":\"ConnectorPlacement.EquallySpacedConnector\",\"uuid\":\"db3b50fc-f4cd-400b-b8f7-b0301a8ba65b\"}],\"packageUris\":[\"http://schema.mathworks.com/mf0/Connector/R2020b\"],\"version\":\"1.0\"}"
      mask Display: image('images/fric_force.png');
  M_clutch : Outport
  wires:
  " "/1 -> Subsystem/1(N), Subsystem1/3(" "), Subsystem2/4(" ")
  Subsystem/1(g(v)) -> Subsystem1/2(g(v))
  Gain3/1 -> Subsystem/2(v), Subsystem1/1(v), Subsystem2/1(v), Scope3/1  "v"
  Gain10/1 -> M_clutch/1  "M_clutch"
  Subsystem2/1(F) -> Gain10/1
  Subsystem1/1(z_dot) -> Subsystem2/2(z_dot), Scope2/2
  Subsystem1/2(z) -> Subsystem2/3(z), Scope2/1
  delta_w/1 -> Gain3/1

== system simulation_upgrade/DRIVETRAIN/Transmission/Gearbox/DCT/Stage_2.1/Nothing ==
  Torque_in : Inport
  Speed_fdbk : Inport  Port=2
  Torque_out : Outport
  Speed_out : Outport  Port=2
  wires:
  Torque_in/1 -> Torque_out/1  "T_Rotor"
  Speed_fdbk/1 -> Speed_out/1

== system simulation_upgrade/DRIVETRAIN/Transmission/Gearbox/DCT/Stage_2.1/Spur ==
  Torque_in : Inport
  Speed_fdbk : Inport  Port=2
  Spur2 : Subsystem  mask{i=Stage2.i1, J1=Stage2.Spur11.J, J2=Stage2.Spur12.J}
      mask prompts: i "Ratio"; J1 "Input_Gear_Inertia"; J2 "Output_Gear_Inertia"
      settings: PortSchema="{\"entries\":[{\"content\":{\"sides\":[{\"content\":{\"connectorIds\":[\"In1\",\"Out2\"]},\"type\":\"ConnectorPlacement.EquallySpacedRectSide\",\"uuid\":\"898fedf9-82f7-4bc2-bf05-880de36b191d\"},{\"content\":{\"connectorIds\":[\"Out1\",\"In2\"],\"side\":\"RIGHT\"},\"type\":\"ConnectorPlacement.EquallySpacedRectSide\",\"uuid\":\"50317b6c-245f-4bd1-a8cd-7a774957ae86\"},{\"content\":{\"side\":\"TOP\"},\"type\":\"ConnectorPlacement.EquallySpacedRectSide\",\"uuid\":\"ff1de2a1-7305-40d8-9e1f-fd0fa1e7d830\"}]},\"type\":\"ConnectorPlacement.EquallySpacedConnector\",\"uuid\":\"6ce82d73-f3da-4f59-9039-464a6ef3e9c5\"}],\"packageUris\":[\"http://schema.mathworks.com/mf0/Connector/R2020b\"],\"version\":\"1.0\"}"
  Torque_out : Outport
  Speed_out : Outport  Port=2
  wires:
  Speed_fdbk/1 -> Spur2/2(Speed_fdbk)
  Torque_in/1 -> Spur2/1(Torque_in)
  Spur2/2(phi_dot) -> Speed_out/1
  Spur2/1(Torque_out) -> Torque_out/1

== system simulation_upgrade/DRIVETRAIN/Transmission/Gearbox/DCT/Stage_2.2/Nothing ==
  Torque_in : Inport
  Speed_fdbk : Inport  Port=2
  Torque_out : Outport
  Speed_out : Outport  Port=2
  wires:
  Torque_in/1 -> Torque_out/1  "T_Rotor"
  Speed_fdbk/1 -> Speed_out/1

== system simulation_upgrade/DRIVETRAIN/Transmission/Gearbox/DCT/Stage_2.2/Spur ==
  Torque_in : Inport
  Speed_fdbk : Inport  Port=2
  Spur2 : Subsystem  mask{i=Stage2.i2, J1=Stage2.Spur21.J, J2=Stage2.Spur22.J}
      mask prompts: i "Ratio"; J1 "Input_Gear_Inertia"; J2 "Output_Gear_Inertia"
      settings: PortSchema="{\"entries\":[{\"content\":{\"sides\":[{\"content\":{\"connectorIds\":[\"In1\",\"Out2\"]},\"type\":\"ConnectorPlacement.EquallySpacedRectSide\",\"uuid\":\"898fedf9-82f7-4bc2-bf05-880de36b191d\"},{\"content\":{\"connectorIds\":[\"Out1\",\"In2\"],\"side\":\"RIGHT\"},\"type\":\"ConnectorPlacement.EquallySpacedRectSide\",\"uuid\":\"50317b6c-245f-4bd1-a8cd-7a774957ae86\"},{\"content\":{\"side\":\"TOP\"},\"type\":\"ConnectorPlacement.EquallySpacedRectSide\",\"uuid\":\"ff1de2a1-7305-40d8-9e1f-fd0fa1e7d830\"}]},\"type\":\"ConnectorPlacement.EquallySpacedConnector\",\"uuid\":\"6ce82d73-f3da-4f59-9039-464a6ef3e9c5\"}],\"packageUris\":[\"http://schema.mathworks.com/mf0/Connector/R2020b\"],\"version\":\"1.0\"}"
  Torque_out : Outport
  Speed_out : Outport  Port=2
  wires:
  Torque_in/1 -> Spur2/1(Torque_in)
  Spur2/2(phi_dot) -> Speed_out/1
  Spur2/1(Torque_out) -> Torque_out/1
  Speed_fdbk/1 -> Spur2/2(Speed_fdbk)

== system simulation_upgrade/DRIVETRAIN/Transmission/Gearbox/DCT/Stage_3/Nothing ==
  Torque_in : Inport
  Speed_fdbk : Inport  Port=2
  Torque_out : Outport
  Speed_out : Outport  Port=2
  wires:
  Speed_fdbk/1 -> Speed_out/1
  Torque_in/1 -> Torque_out/1

== system simulation_upgrade/DRIVETRAIN/Transmission/Gearbox/DCT/Stage_3/Spur ==
  Torque_in : Inport
  Speed_fdbk : Inport  Port=2
  Shaft : Subsystem  mask{J=Shaft.J}
      mask prompts: J "Inertia_kgm^2"
      settings: PortSchema="{\"entries\":[{\"content\":{\"sides\":[{\"content\":{\"connectorIds\":[\"In1\",\"Out2\"]},\"type\":\"ConnectorPlacement.EquallySpacedRectSide\",\"uuid\":\"898fedf9-82f7-4bc2-bf05-880de36b191d\"},{\"content\":{\"connectorIds\":[\"Out1\",\"In2\"],\"side\":\"RIGHT\"},\"type\":\"ConnectorPlacement.EquallySpacedRectSide\",\"uuid\":\"50317b6c-245f-4bd1-a8cd-7a774957ae86\"},{\"content\":{\"side\":\"TOP\"},\"type\":\"ConnectorPlacement.EquallySpacedRectSide\",\"uuid\":\"ff1de2a1-7305-40d8-9e1f-fd0fa1e7d830\"}]},\"type\":\"ConnectorPlacement.EquallySpacedConnector\",\"uuid\":\"6ce82d73-f3da-4f59-9039-464a6ef3e9c5\"}],\"packageUris\":[\"http://schema.mathworks.com/mf0/Connector/R2020b\"],\"version\":\"1.0\"}"
  Spur3 : Subsystem  mask{i=Stage3.i, J1=Stage3.Spur1.J, J2=Stage3.Spur2.J}
      mask prompts: i "Ratio"; J1 "Input_Gear_Inertia"; J2 "Output_Gear_Inertia"
      settings: PortSchema="{\"entries\":[{\"content\":{\"sides\":[{\"content\":{\"connectorIds\":[\"In1\",\"Out2\"]},\"type\":\"ConnectorPlacement.EquallySpacedRectSide\",\"uuid\":\"898fedf9-82f7-4bc2-bf05-880de36b191d\"},{\"content\":{\"connectorIds\":[\"Out1\",\"In2\"],\"side\":\"RIGHT\"},\"type\":\"ConnectorPlacement.EquallySpacedRectSide\",\"uuid\":\"50317b6c-245f-4bd1-a8cd-7a774957ae86\"},{\"content\":{\"side\":\"TOP\"},\"type\":\"ConnectorPlacement.EquallySpacedRectSide\",\"uuid\":\"ff1de2a1-7305-40d8-9e1f-fd0fa1e7d830\"}]},\"type\":\"ConnectorPlacement.EquallySpacedConnector\",\"uuid\":\"6ce82d73-f3da-4f59-9039-464a6ef3e9c5\"}],\"packageUris\":[\"http://schema.mathworks.com/mf0/Connector/R2020b\"],\"version\":\"1.0\"}"
  Torque_out : Outport
  Speed_out : Outport  Port=2
  wires:
  Speed_fdbk/1 -> Spur3/2(Speed_fdbk)
  Spur3/2(phi_dot) -> Shaft/2(Speed_fdbk)
  Spur3/1(Torque_out) -> Torque_out/1
  Torque_in/1 -> Shaft/1(Torque_in)
  Shaft/2(phi_dot) -> Speed_out/1
  Shaft/1(Torque_out) -> Spur3/1(Torque_in)

== system simulation_upgrade/DRIVETRAIN/Transmission/Gearbox/TDT/Stage_1/Nothing ==
  Torque_in : Inport
  Speed_fdbk : Inport  Port=2
  Torque_out : Outport
  Speed_out : Outport  Port=2
  wires:
  Torque_in/1 -> Torque_out/1
  Speed_fdbk/1 -> Speed_out/1

== system simulation_upgrade/DRIVETRAIN/Transmission/Gearbox/TDT/Stage_1/Spur ==
  Torque_in : Inport
  Speed_fdbk : Inport  Port=2
  Shaft1 : Subsystem  mask{J=Shaft.J}
      mask prompts: J "Inertia_kgm^2"
      settings: PortSchema="{\"entries\":[{\"content\":{\"sides\":[{\"content\":{\"connectorIds\":[\"In1\",\"Out2\"]},\"type\":\"ConnectorPlacement.EquallySpacedRectSide\",\"uuid\":\"898fedf9-82f7-4bc2-bf05-880de36b191d\"},{\"content\":{\"connectorIds\":[\"Out1\",\"In2\"],\"side\":\"RIGHT\"},\"type\":\"ConnectorPlacement.EquallySpacedRectSide\",\"uuid\":\"50317b6c-245f-4bd1-a8cd-7a774957ae86\"},{\"content\":{\"side\":\"TOP\"},\"type\":\"ConnectorPlacement.EquallySpacedRectSide\",\"uuid\":\"ff1de2a1-7305-40d8-9e1f-fd0fa1e7d830\"}]},\"type\":\"ConnectorPlacement.EquallySpacedConnector\",\"uuid\":\"6ce82d73-f3da-4f59-9039-464a6ef3e9c5\"}],\"packageUris\":[\"http://schema.mathworks.com/mf0/Connector/R2020b\"],\"version\":\"1.0\"}"
  Spur1 : Subsystem  mask{i=Stage1.i, J1=Stage1.Spur1.J, J2=Stage1.Spur2.J}
      mask prompts: i "Ratio"; J1 "Input_Gear_Inertia"; J2 "Output_Gear_Inertia"
      settings: PortSchema="{\"entries\":[{\"content\":{\"sides\":[{\"content\":{\"connectorIds\":[\"In1\",\"Out2\"]},\"type\":\"ConnectorPlacement.EquallySpacedRectSide\",\"uuid\":\"898fedf9-82f7-4bc2-bf05-880de36b191d\"},{\"content\":{\"connectorIds\":[\"Out1\",\"In2\"],\"side\":\"RIGHT\"},\"type\":\"ConnectorPlacement.EquallySpacedRectSide\",\"uuid\":\"50317b6c-245f-4bd1-a8cd-7a774957ae86\"},{\"content\":{\"side\":\"TOP\"},\"type\":\"ConnectorPlacement.EquallySpacedRectSide\",\"uuid\":\"ff1de2a1-7305-40d8-9e1f-fd0fa1e7d830\"}]},\"type\":\"ConnectorPlacement.EquallySpacedConnector\",\"uuid\":\"6ce82d73-f3da-4f59-9039-464a6ef3e9c5\"}],\"packageUris\":[\"http://schema.mathworks.com/mf0/Connector/R2020b\"],\"version\":\"1.0\"}"
  Torque_out : Outport
  Speed_out : Outport  Port=2
  wires:
  Speed_fdbk/1 -> Shaft1/2(Speed_fdbk)
  Torque_in/1 -> Spur1/1(Torque_in)  "T_Rotor"
  Shaft1/1(Torque_out) -> Torque_out/1  "T_Gear_2"
  Spur1/2(phi_dot) -> Speed_out/1
  Shaft1/2(phi_dot) -> Spur1/2(Speed_fdbk)
  Spur1/1(Torque_out) -> Shaft1/1(Torque_in)

== system simulation_upgrade/DRIVETRAIN/Transmission/Gearbox/TDT/Stage_2.1/Nothing ==
  Torque_in : Inport
  Speed_fdbk : Inport  Port=2
  Torque_out : Outport
  Speed_out : Outport  Port=2
  wires:
  Torque_in/1 -> Torque_out/1  "T_Rotor"
  Speed_fdbk/1 -> Speed_out/1

== system simulation_upgrade/DRIVETRAIN/Transmission/Gearbox/TDT/Stage_2.1/Spur ==
  Torque_in : Inport
  Speed_fdbk : Inport  Port=2
  Shaft1 : Subsystem  mask{J=Shaft.J}
      mask prompts: J "Inertia_kgm^2"
      settings: PortSchema="{\"entries\":[{\"content\":{\"sides\":[{\"content\":{\"connectorIds\":[\"In1\",\"Out2\"]},\"type\":\"ConnectorPlacement.EquallySpacedRectSide\",\"uuid\":\"898fedf9-82f7-4bc2-bf05-880de36b191d\"},{\"content\":{\"connectorIds\":[\"Out1\",\"In2\"],\"side\":\"RIGHT\"},\"type\":\"ConnectorPlacement.EquallySpacedRectSide\",\"uuid\":\"50317b6c-245f-4bd1-a8cd-7a774957ae86\"},{\"content\":{\"side\":\"TOP\"},\"type\":\"ConnectorPlacement.EquallySpacedRectSide\",\"uuid\":\"ff1de2a1-7305-40d8-9e1f-fd0fa1e7d830\"}]},\"type\":\"ConnectorPlacement.EquallySpacedConnector\",\"uuid\":\"6ce82d73-f3da-4f59-9039-464a6ef3e9c5\"}],\"packageUris\":[\"http://schema.mathworks.com/mf0/Connector/R2020b\"],\"version\":\"1.0\"}"
  Spur2 : Subsystem  mask{i=Stage2.i1, J1=Stage2.Spur11.J, J2=Stage2.Spur12.J}
      mask prompts: i "Ratio"; J1 "Input_Gear_Inertia"; J2 "Output_Gear_Inertia"
      settings: PortSchema="{\"entries\":[{\"content\":{\"sides\":[{\"content\":{\"connectorIds\":[\"In1\",\"Out2\"]},\"type\":\"ConnectorPlacement.EquallySpacedRectSide\",\"uuid\":\"898fedf9-82f7-4bc2-bf05-880de36b191d\"},{\"content\":{\"connectorIds\":[\"Out1\",\"In2\"],\"side\":\"RIGHT\"},\"type\":\"ConnectorPlacement.EquallySpacedRectSide\",\"uuid\":\"50317b6c-245f-4bd1-a8cd-7a774957ae86\"},{\"content\":{\"side\":\"TOP\"},\"type\":\"ConnectorPlacement.EquallySpacedRectSide\",\"uuid\":\"ff1de2a1-7305-40d8-9e1f-fd0fa1e7d830\"}]},\"type\":\"ConnectorPlacement.EquallySpacedConnector\",\"uuid\":\"6ce82d73-f3da-4f59-9039-464a6ef3e9c5\"}],\"packageUris\":[\"http://schema.mathworks.com/mf0/Connector/R2020b\"],\"version\":\"1.0\"}"
  Torque_out : Outport
  Speed_out : Outport  Port=2
  wires:
  Speed_fdbk/1 -> Shaft1/2(Speed_fdbk)
  Shaft1/1(Torque_out) -> Torque_out/1  "T_Gear_4"
  Torque_in/1 -> Spur2/1(Torque_in)
  Spur2/2(phi_dot) -> Speed_out/1
  Shaft1/2(phi_dot) -> Spur2/2(Speed_fdbk)
  Spur2/1(Torque_out) -> Shaft1/1(Torque_in)

== system simulation_upgrade/DRIVETRAIN/Transmission/Gearbox/TDT/Stage_2.2/Nothing ==
  Torque_in : Inport
  Speed_fdbk : Inport  Port=2
  Torque_out : Outport
  Speed_out : Outport  Port=2
  wires:
  Torque_in/1 -> Torque_out/1  "T_Rotor"
  Speed_fdbk/1 -> Speed_out/1

== system simulation_upgrade/DRIVETRAIN/Transmission/Gearbox/TDT/Stage_2.2/Spur ==
  Torque_in : Inport
  Speed_fdbk : Inport  Port=2
  Shaft1 : Subsystem  mask{J=Shaft.J}
      mask prompts: J "Inertia_kgm^2"
      settings: PortSchema="{\"entries\":[{\"content\":{\"sides\":[{\"content\":{\"connectorIds\":[\"In1\",\"Out2\"]},\"type\":\"ConnectorPlacement.EquallySpacedRectSide\",\"uuid\":\"898fedf9-82f7-4bc2-bf05-880de36b191d\"},{\"content\":{\"connectorIds\":[\"Out1\",\"In2\"],\"side\":\"RIGHT\"},\"type\":\"ConnectorPlacement.EquallySpacedRectSide\",\"uuid\":\"50317b6c-245f-4bd1-a8cd-7a774957ae86\"},{\"content\":{\"side\":\"TOP\"},\"type\":\"ConnectorPlacement.EquallySpacedRectSide\",\"uuid\":\"ff1de2a1-7305-40d8-9e1f-fd0fa1e7d830\"}]},\"type\":\"ConnectorPlacement.EquallySpacedConnector\",\"uuid\":\"6ce82d73-f3da-4f59-9039-464a6ef3e9c5\"}],\"packageUris\":[\"http://schema.mathworks.com/mf0/Connector/R2020b\"],\"version\":\"1.0\"}"
  Spur2 : Subsystem  mask{i=Stage2.i2, J1=Stage2.Spur21.J, J2=Stage2.Spur22.J}
      mask prompts: i "Ratio"; J1 "Input_Gear_Inertia"; J2 "Output_Gear_Inertia"
      settings: PortSchema="{\"entries\":[{\"content\":{\"sides\":[{\"content\":{\"connectorIds\":[\"In1\",\"Out2\"]},\"type\":\"ConnectorPlacement.EquallySpacedRectSide\",\"uuid\":\"898fedf9-82f7-4bc2-bf05-880de36b191d\"},{\"content\":{\"connectorIds\":[\"Out1\",\"In2\"],\"side\":\"RIGHT\"},\"type\":\"ConnectorPlacement.EquallySpacedRectSide\",\"uuid\":\"50317b6c-245f-4bd1-a8cd-7a774957ae86\"},{\"content\":{\"side\":\"TOP\"},\"type\":\"ConnectorPlacement.EquallySpacedRectSide\",\"uuid\":\"ff1de2a1-7305-40d8-9e1f-fd0fa1e7d830\"}]},\"type\":\"ConnectorPlacement.EquallySpacedConnector\",\"uuid\":\"6ce82d73-f3da-4f59-9039-464a6ef3e9c5\"}],\"packageUris\":[\"http://schema.mathworks.com/mf0/Connector/R2020b\"],\"version\":\"1.0\"}"
  Torque_out : Outport
  Speed_out : Outport  Port=2
  wires:
  Torque_in/1 -> Spur2/1(Torque_in)
  Shaft1/1(Torque_out) -> Torque_out/1  "T_Gear_4"
  Speed_fdbk/1 -> Shaft1/2(Speed_fdbk)
  Spur2/2(phi_dot) -> Speed_out/1
  Shaft1/2(phi_dot) -> Spur2/2(Speed_fdbk)
  Spur2/1(Torque_out) -> Shaft1/1(Torque_in)

== system simulation_upgrade/DRIVETRAIN/Transmission/Gearbox/TDT/Stage_3/Nothing ==
  Torque_in : Inport
  Speed_fdbk : Inport  Port=2
  Torque_out : Outport
  Speed_out : Outport  Port=2
  wires:
  Torque_in/1 -> Torque_out/1
  Speed_fdbk/1 -> Speed_out/1

== system simulation_upgrade/DRIVETRAIN/Transmission/Gearbox/TDT/Stage_3/Spur ==
  Torque_in : Inport
  Speed_fdbk : Inport  Port=2
  Spur3 : Subsystem  mask{i=Stage3.i, J1=Stage3.Spur1.J, J2=Stage3.Spur2.J}
      mask prompts: i "Ratio"; J1 "Input_Gear_Inertia"; J2 "Output_Gear_Inertia"
      settings: PortSchema="{\"entries\":[{\"content\":{\"sides\":[{\"content\":{\"connectorIds\":[\"In1\",\"Out2\"]},\"type\":\"ConnectorPlacement.EquallySpacedRectSide\",\"uuid\":\"898fedf9-82f7-4bc2-bf05-880de36b191d\"},{\"content\":{\"connectorIds\":[\"Out1\",\"In2\"],\"side\":\"RIGHT\"},\"type\":\"ConnectorPlacement.EquallySpacedRectSide\",\"uuid\":\"50317b6c-245f-4bd1-a8cd-7a774957ae86\"},{\"content\":{\"side\":\"TOP\"},\"type\":\"ConnectorPlacement.EquallySpacedRectSide\",\"uuid\":\"ff1de2a1-7305-40d8-9e1f-fd0fa1e7d830\"}]},\"type\":\"ConnectorPlacement.EquallySpacedConnector\",\"uuid\":\"6ce82d73-f3da-4f59-9039-464a6ef3e9c5\"}],\"packageUris\":[\"http://schema.mathworks.com/mf0/Connector/R2020b\"],\"version\":\"1.0\"}"
  Torque_out : Outport
  Speed_out : Outport  Port=2
  wires:
  Torque_in/1 -> Spur3/1(Torque_in)
  Spur3/1(Torque_out) -> Torque_out/1
  Spur3/2(phi_dot) -> Speed_out/1
  Speed_fdbk/1 -> Spur3/2(Speed_fdbk)

== system simulation_upgrade/DRIVETRAIN/Transmission/Gearbox/AMT/Clutch/Clutch1/Subsystem ==
  N : Inport
  v : Inport  Port=2
  Abs : Abs  SaturateOnIntegerOverflow=off
  Constant1 : Constant  Value=vs
  Divide1 : Product  Inputs=/*
  Divide2 : Product  Inputs=/*
  Exp : Math
  Gain1 : Gain  Gain=n_surfaces
  Gain4 : Gain  Gain=mi_s
  Gain5 : Gain  Gain=1/sigma0
  Gain6 : Gain  Gain=mi_c
  Gain7 : Gain  Gain=N_clutch*2
  Square : Math  Operator=square
  Sum4 : Sum  Inputs=+|+
  Sum5 : Sum  Inputs=|+-
  g(v) : Outport
  wires:
  Gain1/1 -> Gain4/1, Gain6/1
  Gain4/1 -> Sum5/1  "Fs"
  Abs/1 -> Gain7/1
  v/1 -> Divide1/2
  N/1 -> Abs/1
  Gain5/1 -> g(v)/1  "g(v)"
  Square/1 -> Exp/1
  Divide1/1 -> Square/1
  Constant1/1 -> Divide1/1
  Gain7/1 -> Gain1/1  "Fn"
  Exp/1 -> Divide2/1
  Gain6/1 -> Sum5/2, Sum4/2  "Fc"
  Divide2/1 -> Sum4/1
  Sum5/1 -> Divide2/2
  Sum4/1 -> Gain5/1

== system simulation_upgrade/DRIVETRAIN/Transmission/Gearbox/AMT/Clutch/Clutch1/Subsystem1 ==
  v : Inport
  g(v) : Inport  Port=2
  In1 : Inport  Port=3
  Abs1 : Abs  SaturateOnIntegerOverflow=off
  Divide : Product  Inputs=*/
  Integrator : Integrator
  Product2 : Product
  Saturation : Saturate  UpperLimit=inf  LowerLimit=0.01
  Sum2 : Sum  Inputs=|+-
  Switch : Switch  Criteria=u2 ~= 0  SaturateOnIntegerOverflow=off  InputSameDT=off
  z_dot : Outport
  z : Outport  Port=2
  wires:
  In1/1 -> Switch/2, Switch/3
  g(v)/1 -> Saturation/1
  Product2/1 -> Sum2/2
  Abs1/1 -> Divide/1
  Saturation/1 -> Divide/2
  Sum2/1 -> z_dot/1, Integrator/1  "z_dot"
  Switch/1 -> Abs1/1, Sum2/1
  Divide/1 -> Product2/1
  Integrator/1 -> Product2/2, z/1  "z"
  v/1 -> Switch/1
